simulink library "slctrlextras"  (Simulink 6.0)
settings: Solver=ode45  SolverMode=SingleTasking  StartTime=0.0  StopTime=10.0  RelTol=1e-3
libraries: slctrlblks x1
settings Model: Creator=jglass  LastModifiedBy=jglass
settings DataIOCC: SignalLoggingName=logsOut
settings OptimizationCC: BooleanDataType=off
settings DebuggingCC: CheckExecutionContextPreStartOutputMsg=on  CheckExecutionContextRuntimeOutputMsg=on  SolverPrmCheckMsg=none
settings HardwareCC: TargetUnknown=on
settings GRTTargetCC: UtilityFuncGeneration=Automatic  LifeSpan=inf
settings SFSimCC: SFSimApplyToAllLibs=on  SFSimBuildMode=Incremental

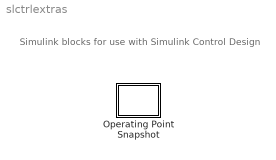
== system slctrlextras ==
  note: Simulink blocks for use with Simulink Control Design
  Operating Point Snapshot : Subsystem  EnableExecutionContextPropagation=on  mask(Time Operating Condition Snapshot){SnapshotTimes=[1 2]}
      mask prompts: SnapshotTimes "Operating point snapshot times:"
      mask help: Generate linear models in the base workspace at specific times.
      mask Help: This block calls LINMOD or DLINMOD to create a linear model for the system when the simulation clock reaches the time specified by the LinearizationTime parameter.  No trimming is performed.  The linear model is stored in the base workspace as a structure, along with information about the operating point at which the snapshot was taken.  Multiple snapshots are appended to form an array of structures.
      mask Display: disp(['T=' mat2str(SnapshotTimes)])

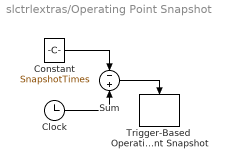
== system slctrlextras/Operating Point Snapshot ==
  Clock : Clock
      settings: Decimation=10
  Constant : Constant  Value=SnapshotTimes
  Sum : Sum  Inputs=-+  SaturateOnIntegerOverflow=on  InputSameDT=on
  Trigger-Based  Operating Point Snapshot : slctrlblks/Trigger-Based  Operating Point Snapshot  TriggerType=rising
  wires:
  Sum/1 -> Trigger-Based  Operating Point Snapshot/Trigger
  Constant/1 -> Sum/1
  Clock/1 -> Sum/2
